simulink model "test_three_phase_lines"  (R2025b)
settings: Solver=VariableStepAuto  StartTime=0.0  StopTime=1  RelTol=1e-3
libraries: ee_lib x13, ee_lib_for_power_systems x9, nesl_utility x7, fl_lib x6
settings Model: SimulationMode=accelerator  Creator=gdudgeon  LastModifiedBy=gdudgeon
settings RTWCC: GPUComputeCapability=3.5

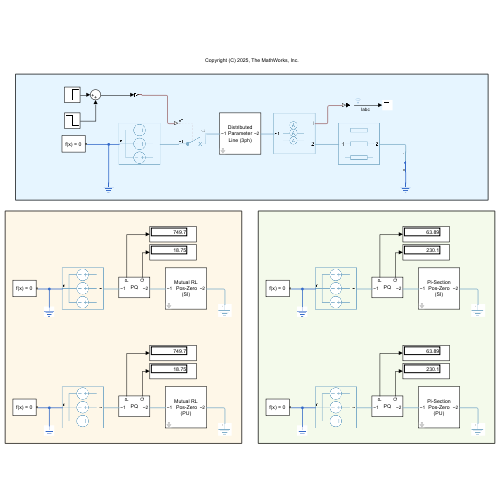
[thumbnail: Simulink's stored preview of the top-level diagram]
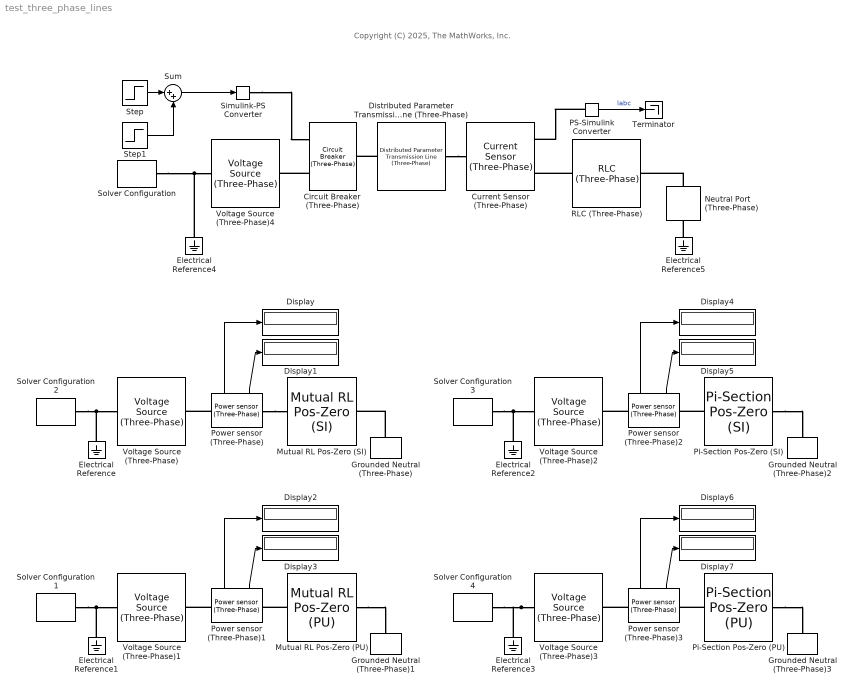
== system test_three_phase_lines ==
  note: Copyright (C) 2025, The MathWorks, Inc.
  Circuit Breaker (Three-Phase) : ee_lib/Switches & Breakers/Circuit Breaker (Three-Phase)  R_closed=1e-6 Ohm  G_open=1e-6 1/Ohm  threshold=0.5 V  breaker_behavior=ee.enum.switches.breakerBehavior.zeroCrossingEnable
      settings: InternalSimscapePortConfiguration="{\"Bottom\":[],\"Left\":[{\"id\":\"vT\",\"label\":\"vT\",\"type\":\"input\"},{\"id\":\"N1\",\"label\":\"~1\",\"type\":\"foundation.electrical.three_phase\"}],\"Right\":[{\"id\":\"N2\",\"label\":\"~2\",\"type\":\"foundation.electrical.three_phase\"}],\"Top\":[]}"
  Current Sensor (Three-Phase) : ee_lib/Sensors & Transducers/Current Sensor (Three-Phase)
  Display{,1..7} (8 alike) : Display
  "Distributed Parameter Transmission Line (Three-Phase) " : ee_lib_for_power_systems/Network Components/Distributed Parameter Transmission Line (Three-Phase)   length=100  Fnom=60  R1_L1_C1=[1e-2 1e-3 15e-9]  R0_L0_C0=[0.2 5e-3 5e-9]  run_time=on
      settings: SourceProductName=Support Library for Power Systems
  Electrical Reference{,1..5} (6 alike) : fl_lib/Electrical/Electrical Elements/Electrical Reference
  Grounded Neutral (Three-Phase){,1..3} (4 alike) : ee_lib/Connectors & References/Grounded Neutral (Three-Phase)
  Mutual RL Pos-Zero (PU) : ee_lib_for_power_systems/Network Components/Mutual RL Pos-Zero (PU)  Pnom_Vnom_Fnom=[1e3 100 60]  R1_L1=[2 0.05]  R0_L0=[4 0.1]  run_time=off
      settings: SourceProductName=Support Library for Power Systems
  Mutual RL Pos-Zero (SI) : ee_lib_for_power_systems/Network Components/Mutual RL Pos-Zero (SI)  R1_L1=[20 0.05*1e3/100/(2*pi*60)]  R0_L0=[40 0.1*1e3/100/(2*pi*60)]  run_time=off
      settings: SourceProductName=Support Library for Power Systems
  Neutral Port (Three-Phase) : ee_lib/Connectors & References/Neutral Port (Three-Phase)  G_parasitic=1e-12 1/Ohm
      settings: InternalSimscapePortConfiguration="{\"Bottom\":[],\"Left\":[{\"id\":\"N\",\"label\":\"~\",\"type\":\"foundation.electrical.three_phase\"}],\"Right\":[{\"id\":\"n\",\"label\":\"n\",\"type\":\"foundation.electrical.electrical\"}],\"Top\":[]}"
  PS-Simulink Converter : nesl_utility/PS-Simulink Converter  PhysicalDomain=network_engine_domain  SubClassName=ps_output  LeftPortType=input  RightPortType=output  PseudoPeriodic=off  Frequencies=[]  VectorFormat=inherit  Unit=inherit  AffineConversion=off
  Pi-Section Pos-Zero (PU) : ee_lib_for_power_systems/Network Components/Pi-Section Pos-Zero (PU)  length=100  Pnom_Vnom_Fnom=[5e6 5e3 60]  R1_L1_C1=[0.02 0.0754 1.885e-4]  R0_L0_C0=[0.1 0.377 1.885e-5]  run_time=on
      settings: SourceProductName=Support Library for Power Systems
  Pi-Section Pos-Zero (SI) : ee_lib_for_power_systems/Network Components/Pi-Section Pos-Zero (SI)  length=100  Fnom=60  R1_L1_C1=[0.1 0.001 1e-7]  R0_L0_C0=[0.5 0.005 1e-8]  run_time=on
      settings: SourceProductName=Support Library for Power Systems
  Power sensor (Three-Phase){,1..3} (4 alike) : ee_lib_for_power_systems/Sense and Measure/Power sensor (Three-Phase)  SystemSampleTime=-1  VariantActivationTime=update diagram  EmptyChoice=off  PassThrough=off  PassThroughVariantControl=(default)  EmptyChoiceVariantControl=(default)  AllowFlexibleInterface=on  Latency=0  AutoFrameSizeCalculation=off
      settings: SourceProductName=Support Library for Power Systems  PortSchema="{\"entries\":[{\"content\":{\"sides\":[{\"content\":{\"connectorIds\":[\"LConn1\"]},\"type\":\"ConnectorPlacement.EquallySpacedRectSide\",\"uuid\":\"d536c57f-d596-4c30-b2f2-ca7a7128ca09\"},{\"content\":{\"connectorIds\":[\"RConn1\"],\"side\":\"RIGHT\"},\"type\":\"ConnectorPlacement.EquallySpacedRectSide\",\"uuid\":\"3e38bcb4-aad6-4c8e-8ba0-f34fad0d941d\"},{\"content\":{\"connectorIds\":[\"Out1\",\"Out2\"],\"side\":\"TOP\"},\"type\":\"ConnectorPlacement.EquallySpacedRectSide\",\"uuid\":\"dbbb5dbf-676f-46fa-997f-a90b77759865\"}]},\"type\":\"ConnectorPlacement.EquallySpacedConnector\",\"uuid\":\"d250c4d3-27c8-4176-913c-392fad876444\"}],\"packageUris\":[\"http://schema.mathworks.com/mf0/Connector/R2020b\"],\"version\":\"1.0\"}"
  RLC (Three-Phase) : ee_lib/Passive/RLC Assemblies/RLC (Three-Phase)  port_option=ee.enum.threePhasePort.composite  component_structure=ee.enum.rlc.structure.R  R=10 Ohm  L=1e-3 H  C=1e-6 F  R_parasitic=0 Ohm  G_parasitic=0 1/Ohm  IL_specify=off  IL_priority=High  IL=[0, 0, 0] A  IL_nominal_specify=off  IL_nominal_value=1  IL_nominal_unit=A  VC_specify=off  VC_priority=High  VC=[0, 0, 0] V  VC_nominal_specify=off  VC_nominal_value=1  VC_nominal_unit=V
      settings: InternalSimscapePortConfiguration="{\"Bottom\":[],\"Left\":[{\"id\":\"N1\",\"label\":\"~1\",\"type\":\"foundation.electrical.three_phase\"}],\"Right\":[{\"id\":\"N2\",\"label\":\"~2\",\"type\":\"foundation.electrical.three_phase\"}],\"Top\":[]}"
  Simulink-PS Converter : nesl_utility/Simulink-PS Converter  PhysicalDomain=network_engine_domain  SubClassName=ps_input  LeftPortType=input  RightPortType=output  PseudoPeriodic=off  Frequencies=[]  NoiseDistribution=none  NoiseParameters=[]  Unit=1  AffineConversion=off  FilteringAndDerivatives=provide  SimscapeFilterOrder=1  InputFilterTimeConstant=0.001  UdotUserProvided=0
  Solver Configuration : nesl_utility/Solver Configuration  PhysicalDomain=network_engine_domain  SubClassName=solver  LeftPortType=input  RightPortType=generic  Tones=[]  Harmonics=[]  SimulateNoise=off  Profile=off  UseLocalSampling=off  EnableSwitchedLinearOptims=on  FrequencyDomain=off  UseCCode=off  RelTol=0.001  AbsTol=0.001  MinStep=1e-09  ToWorkspace=off  RevertToSquareIcSolve=off  NumHomotopyIterations=100  PhasorMode=off  PhasorModeNumHarmonics=1  ConsistencySolver=NEWTON_XTOL_AFTER_FTOL  IndexReductionMethod=DerivativeReplacement  DoDC=off  ResidualTolerance=1e-09  ConsistencyTolSource=GLOBAL  ConsistencyAbsTol=0.001  ConsistencyRelTol=0.001  ConsistencyTolFactor=0.001  UseLocalSolver=on  LocalSolverChoice=NE_BACKWARD_EULER_ADVANCER  ResolveIndetEquations=off  FunctionEvalNumThread=1  LocalSolverSampleTime=5e-5  DoFixedCost=on  MaxNonlinIter=1  MaxModeIter=2  ComputeImpulses=off  ImpulseIterations=2  LinearAlgebra=auto  LinearAlgebraNumThread=0  EquationFormulation=NE_TIME_EF  DelaysMemoryBudget=1024  AutomaticFiltering=off  FilteringTimeConstant=0.001  PartitionStorageMethod=AS_NEEDED  PartitionMemoryBudget=1024  PartitionMethod=ROBUST  MultibodyUseLocalSolver=off  MultibodyLocalSolverChoice=ODE1  MultibodyLocalSolverSampleTime=0.001
  Solver Configuration {1..4} (4 alike) : nesl_utility/Solver Configuration  PhysicalDomain=network_engine_domain  SubClassName=solver  LeftPortType=input  RightPortType=generic  Tones=[]  Harmonics=[]  SimulateNoise=off  Profile=off  UseLocalSampling=off  EnableSwitchedLinearOptims=on  FrequencyDomain=off  UseCCode=off  RelTol=0.001  AbsTol=0.001  MinStep=1e-09  ToWorkspace=off  RevertToSquareIcSolve=off  NumHomotopyIterations=100  PhasorMode=off  PhasorModeNumHarmonics=1  ConsistencySolver=NEWTON_XTOL_AFTER_FTOL  IndexReductionMethod=None  DoDC=off  ResidualTolerance=1e-09  ConsistencyTolSource=GLOBAL  ConsistencyAbsTol=0.001  ConsistencyRelTol=0.001  ConsistencyTolFactor=0.001  UseLocalSolver=on  LocalSolverChoice=NE_PARTITIONING_ADVANCER  ResolveIndetEquations=off  FunctionEvalNumThread=1  LocalSolverSampleTime=50e-6  DoFixedCost=off  MaxNonlinIter=2  MaxModeIter=2  ComputeImpulses=off  ImpulseIterations=2  LinearAlgebra=Sparse  LinearAlgebraNumThread=0  EquationFormulation=NE_TIME_EF  DelaysMemoryBudget=1024  AutomaticFiltering=off  FilteringTimeConstant=0.001  PartitionStorageMethod=AS_NEEDED  PartitionMemoryBudget=1024  PartitionMethod=ROBUST  MultibodyUseLocalSolver=off  MultibodyLocalSolverChoice=ODE1  MultibodyLocalSolverSampleTime=0.001
  Step : Step  Time=0.5  SampleTime=0
  Step1 : Step  Time=0.55  After=-1  SampleTime=0
  Sum : Sum  Inputs=|++
  Terminator : Terminator
  Voltage Source (Three-Phase) : ee_lib/Sources/Voltage Source (Three-Phase)  vline_rms=sqrt(3) * 100 / sqrt(2) V  shift=0 deg  freq=60 Hz  impedance_option=0  SShortCircuit=1e6 A*V  XR=15  R=0.01 Ohm  L=3.97e-4 H  harmonic_option=0  harmonic_orders=[5, 7, 11, 13]  harmonic_ratios=[.1, .1, .1, .1]  G_parasitic=0 1/Ohm  I_specify=off  I_priority=None  I=[0, 0, 0] A  I_nominal_specify=off  I_nominal_value=1  I_nominal_unit=A
  Voltage Source (Three-Phase)1 : ee_lib/Sources/Voltage Source (Three-Phase)  vline_rms=sqrt(3) * 100 / sqrt(2) V  shift=0 deg  freq=60 Hz  impedance_option=0  SShortCircuit=1e6 A*V  XR=15  R=0.01 Ohm  L=3.97e-4 H  harmonic_option=0  harmonic_orders=[5, 7, 11, 13]  harmonic_ratios=[.1, .1, .1, .1]  G_parasitic=0 1/Ohm  I_specify=off  I_priority=None  I=[0, 0, 0] A  I_nominal_specify=off  I_nominal_value=1  I_nominal_unit=A
  Voltage Source (Three-Phase)2 : ee_lib/Sources/Voltage Source (Three-Phase)  vline_rms=100 V  shift=0 deg  freq=60 Hz  impedance_option=0  SShortCircuit=1e6 A*V  XR=15  R=0.01 Ohm  L=3.97e-4 H  harmonic_option=0  harmonic_orders=[5, 7, 11, 13]  harmonic_ratios=[.1, .1, .1, .1]  G_parasitic=0 1/Ohm  I_specify=off  I_priority=None  I=[0, 0, 0] A  I_nominal_specify=off  I_nominal_value=1  I_nominal_unit=A
  Voltage Source (Three-Phase)3 : ee_lib/Sources/Voltage Source (Three-Phase)  vline_rms=100 V  shift=0 deg  freq=60 Hz  impedance_option=0  SShortCircuit=1e6 A*V  XR=15  R=0.01 Ohm  L=3.97e-4 H  harmonic_option=0  harmonic_orders=[5, 7, 11, 13]  harmonic_ratios=[.1, .1, .1, .1]  G_parasitic=0 1/Ohm  I_specify=off  I_priority=None  I=[0, 0, 0] A  I_nominal_specify=off  I_nominal_value=1  I_nominal_unit=A
  Voltage Source (Three-Phase)4 : ee_lib/Sources/Voltage Source (Three-Phase)  vline_rms=1000 V  shift=0 deg  freq=60 Hz  impedance_option=0  SShortCircuit=1e6 A*V  XR=15  R=0.01 Ohm  L=3.97e-4 H  harmonic_option=0  harmonic_orders=[5, 7, 11, 13]  harmonic_ratios=[.1, .1, .1, .1]  G_parasitic=0 1/Ohm  I_specify=off  I_priority=None  I=[0, 0, 0] A  I_nominal_specify=off  I_nominal_value=1  I_nominal_unit=A
  wires:
  Power sensor (Three-Phase)/1 -> Display/1
  Power sensor (Three-Phase)/2 -> Display1/1
  Power sensor (Three-Phase)1/2 -> Display3/1
  Power sensor (Three-Phase)1/1 -> Display2/1
  Power sensor (Three-Phase)2/2 -> Display5/1
  Power sensor (Three-Phase)2/1 -> Display4/1
  Power sensor (Three-Phase)3/1 -> Display6/1
  Power sensor (Three-Phase)3/2 -> Display7/1
  Step/1 -> Sum/1
  Step1/1 -> Sum/2
  PS-Simulink Converter/1 -> Terminator/1  "Iabc"
  Sum/1 -> Simulink-PS Converter/1
  connections:
  Electrical Reference/LConn1 -- Solver Configuration 2/RConn1 -- Voltage Source (Three-Phase)/LConn1
  Grounded Neutral (Three-Phase)/LConn1 -- Mutual RL Pos-Zero (SI)/RConn1
  Power sensor (Three-Phase)/LConn1 -- Voltage Source (Three-Phase)/RConn1
  Power sensor (Three-Phase)/RConn1 -- Mutual RL Pos-Zero (SI)/LConn1
  Solver Configuration 1/RConn1 -- Voltage Source (Three-Phase)1/LConn1 -- Electrical Reference1/LConn1
  Mutual RL Pos-Zero (PU)/LConn1 -- Power sensor (Three-Phase)1/RConn1
  Mutual RL Pos-Zero (PU)/RConn1 -- Grounded Neutral (Three-Phase)1/LConn1
  Power sensor (Three-Phase)1/LConn1 -- Voltage Source (Three-Phase)1/RConn1
  Solver Configuration 3/RConn1 -- Voltage Source (Three-Phase)2/LConn1 -- Electrical Reference2/LConn1
  Pi-Section Pos-Zero (SI)/LConn1 -- Power sensor (Three-Phase)2/RConn1
  Pi-Section Pos-Zero (SI)/RConn1 -- Grounded Neutral (Three-Phase)2/LConn1
  Power sensor (Three-Phase)2/LConn1 -- Voltage Source (Three-Phase)2/RConn1
  Voltage Source (Three-Phase)3/LConn1 -- Solver Configuration 4/RConn1 -- Electrical Reference3/LConn1
  Pi-Section Pos-Zero (PU)/RConn1 -- Grounded Neutral (Three-Phase)3/LConn1
  Pi-Section Pos-Zero (PU)/LConn1 -- Power sensor (Three-Phase)3/RConn1
  Power sensor (Three-Phase)3/LConn1 -- Voltage Source (Three-Phase)3/RConn1
  Solver Configuration/RConn1 -- Electrical Reference4/LConn1 -- Voltage Source (Three-Phase)4/LConn1
  Circuit Breaker (Three-Phase)/LConn2 -- Voltage Source (Three-Phase)4/RConn1
  RLC (Three-Phase)/LConn1 -- Current Sensor (Three-Phase)/RConn2
  PS-Simulink Converter/LConn1 -- Current Sensor (Three-Phase)/RConn1
  "Distributed Parameter Transmission Line (Three-Phase) "/RConn1 -- Current Sensor (Three-Phase)/LConn1
  Neutral Port (Three-Phase)/LConn1 -- RLC (Three-Phase)/RConn1
  Simulink-PS Converter/RConn1 -- Circuit Breaker (Three-Phase)/LConn1
  "Distributed Parameter Transmission Line (Three-Phase) "/LConn1 -- Circuit Breaker (Three-Phase)/RConn1
  Electrical Reference5/LConn1 -- Neutral Port (Three-Phase)/RConn1
